simulink model "maglev"  (Simulink 9.1)
settings: Solver=ode45  StartTime=0.0  StopTime=9  MaxStep=T/10  RelTol=1e-3  EnableMultiTasking=on
StopFcn:
  | geragraficos
values from neighbouring files (symbols this model uses):
  dt = 0.001    [kalman_function.m]    (also in q6.m = 0.005)
  Gcd = 60*tf([1/alphae 1-1/alphae-exp(-tempo/(alphae*T))],[1 -exp(-tempo/(alphae*T))], tempo)    [q6.m]
  h_sig = 0.002/3    (= 0.000666666666667)    [q6.m]
  P0 = [0 0; 0 0]    [q6.m]
  x0 = [href;0]    [q6.m]
undefined symbols (not defined in the file or in its folder): sigbuilder_block
settings Model: Creator=cairo  LastModifiedBy=Avell
settings DataIOCC: LimitDataPoints=on  SignalLoggingSaveFormat=ModelDataLogs
settings OptimizationCC: ExpressionDepthLimit=2147483647  InitFltsAndDblsToZero=on
settings DebuggingCC: SaveWithParameterizedLinksMsg=none  SignalResolutionControl=TryResolveAllWithWarning  SolverPrmCheckMsg=warning  MultiTaskDSMMsg=warning  MultiTaskCondExecSysMsg=none  FcnCallInpInsideContextMsg=warning  StateNameClashWarn=warning
settings GRTTargetCC: TargetFcnLib=ansi_tfl_tmw.mat  GeneratePreprocessorConditionals=Disable all

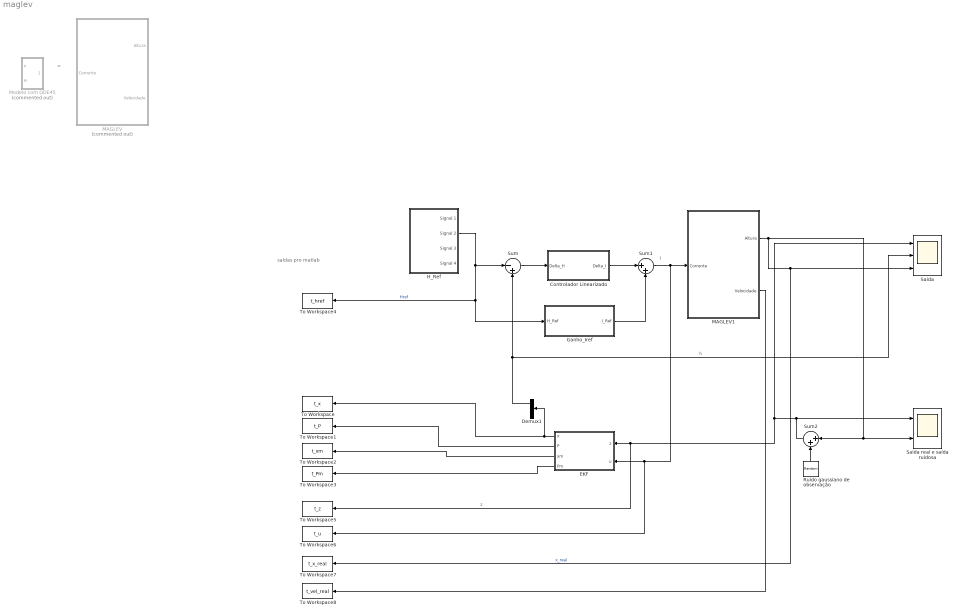
== system maglev ==
  note: saídas pro matlab
  note: =
  note: I
  Controlador Linearizado : Subsystem  mask(Controlador em avanço + termo integrador){}
  Demux1 : Demux  Outputs=2
  EKF : Subsystem
  Ganho_Iref : Subsystem  mask(Cálculo da corrente de referência (I_Ref) a partir da altura de referência (H_Ref)){Kb=0.12e-3, M=21.2e-3, g=9.8}
      mask prompts: Kb "Constante da bobina (Nm^2/A^2)"; M "Massa (kg)"; g "Gravidade (m/s^2)"
  H_Ref : Subsystem  Tag=STV Subsys  LoadFcn=sigbuilder_block('load');  StartFcn=sigbuilder_block('start');  StopFcn=sigbuilder_block('stop');  ClipboardFcn=sigbuilder_block('clipboard');  mask(Sigbuilder block){tuvar=[0:10]}
      mask help: Sigbuilder GUI
      mask init:
      | if ~strcmp(get_param(bdroot(gcbh),'SimulationStatus'),'stopped') tuvar = sigbuilder_block('maskInit'); end
      settings: CopyFcn=sigbuilder_block('copy');  DeleteFcn=sigbuilder_block('delete');  ModelCloseFcn=sigbuilder_block('modelClose');  PreSaveFcn=sigbuilder_block('preSave');  PauseFcn=sigbuilder_block('pause')  ContinueFcn=sigbuilder_block('continue')  NameChangeFcn=sigbuilder_block('namechange');  OpenFcn=sigbuilder_block('open',[0 0 1390.5 752.25 ]);  CloseFcn=sigbuilder_block('close');
      mask Display: plot(0, 0, 100, 100,[2, 2, 32, 32, 2], [68, 8, 8, 68, 68],[32, 2], [38, 38], [32, 19, 2],[53, 60, 44], [32, 17, 17, 2],[16, 16, 31, 31]);txt = getActiveGroup(gcbh);text(2, 100, txt,'verticalAlignment', 'top');
  MAGLEV : Subsystem  Commented=on  mask{Kb=0.12e-3, M=21.2e-3, g=9.8, x1_0=0.030, x2_0=0}
      mask prompts: Kb "Constante da bobina (Nm^2/A^2)"; M "Massa (kg)"; g "Gravidade (m/s^2)"; x1_0 "Altura inicial (m)"; x2_0 "Velocidade Inicial (m/s)"
      mask help: Modelo do Sistema de Levitação Magnética
      mask Display: image(imread('maglev_fig.jpg'),[0,0,350/2.5,525/2.5]);
  MAGLEV1 : Subsystem  mask{Kb=0.12e-3, M=21.2e-3, g=9.8, x1_0=0.030, x2_0=0}
      mask prompts: Kb "Constante da bobina (Nm^2/A^2)"; M "Massa (kg)"; g "Gravidade (m/s^2)"; x1_0 "Altura inicial (m)"; x2_0 "Velocidade Inicial (m/s)"
      mask help: Modelo do Sistema de Levitação Magnética
      mask Display: image(imread('maglev_fig.jpg'),[0,0,350/2.5,525/2.5]);
  Modelo com ODE45 : Subsystem  Commented=on
  Ruido gaussiano de observação : RandomNumber  Variance=h_sig^2  SampleTime=dt
  Saida : Scope  NumInputPorts=3
  Saida real e saída ruidosa : Scope  NumInputPorts=2
  Sum : Sum  Inputs=|-+
  Sum1 : Sum  Inputs=|++
  Sum2 : Sum  Inputs=|++
  To Workspace : ToWorkspace  VariableName=t_x  SaveFormat=Timeseries  SampleTime=-1
  To Workspace1 : ToWorkspace  VariableName=t_P  SaveFormat=Timeseries  SampleTime=-1
  To Workspace2 : ToWorkspace  VariableName=t_xm  SaveFormat=Timeseries  SampleTime=-1
  To Workspace3 : ToWorkspace  VariableName=t_Pm  SaveFormat=Timeseries  SampleTime=-1
  To Workspace4 : ToWorkspace  VariableName=t_href  SaveFormat=Timeseries  SampleTime=-1
  To Workspace5 : ToWorkspace  VariableName=t_z  SaveFormat=Timeseries  SampleTime=-1
  To Workspace6 : ToWorkspace  VariableName=t_u  SaveFormat=Timeseries  SampleTime=-1
  To Workspace7 : ToWorkspace  VariableName=t_x_real  SaveFormat=Timeseries  SampleTime=-1
  To Workspace8 : ToWorkspace  VariableName=t_vel_real  SaveFormat=Timeseries  SampleTime=-1
  wires:
  Ganho_Iref/1(I_Ref) -> Sum1/2
  Sum/1 -> Controlador Linearizado/1(Delta_H)
  Controlador Linearizado/1(Delta_I) -> Sum1/1
  H_Ref/2(Signal 2) -> Ganho_Iref/1(H_Ref), To Workspace4/1, Sum/1  "Href"
  Ruido gaussiano de observação/1 -> Sum2/2
  Sum2/1 -> To Workspace5/1, EKF/1(z), Saida/1, Saida real e saída ruidosa/1  "z"
  MAGLEV1/1(Altura) -> Saida real e saída ruidosa/2, Sum2/1, To Workspace7/1, Saida/3  "x_real"
  Sum1/1 -> To Workspace6/1, EKF/2(u), MAGLEV1/1(Corrente)
  EKF/1(x) -> To Workspace/1, Demux1/1
  Demux1/1 -> Saida/2, Sum/2  "h"
  EKF/2(P) -> To Workspace1/1
  EKF/3(xm) -> To Workspace2/1
  EKF/4(Pm) -> To Workspace3/1
  MAGLEV1/2(Velocidade) -> To Workspace8/1

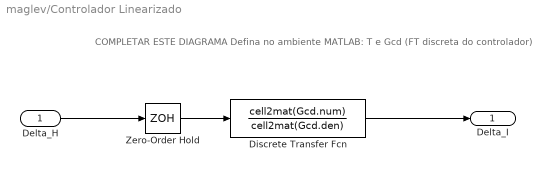
== system maglev/Controlador Linearizado ==
  note: COMPLETAR ESTE DIAGRAMA
      | Defina no ambiente MATLAB: T e Gcd (FT discreta do controlador)
  Delta_H : Inport
  Discrete Transfer Fcn : DiscreteTransferFcn  Numerator=cell2mat(Gcd.num)  Denominator=cell2mat(Gcd.den)
  Zero-Order Hold : ZeroOrderHold  SampleTime=dt
  Delta_I : Outport
  wires:
  Delta_H/1 -> Zero-Order Hold/1
  Discrete Transfer Fcn/1 -> Delta_I/1
  Zero-Order Hold/1 -> Discrete Transfer Fcn/1

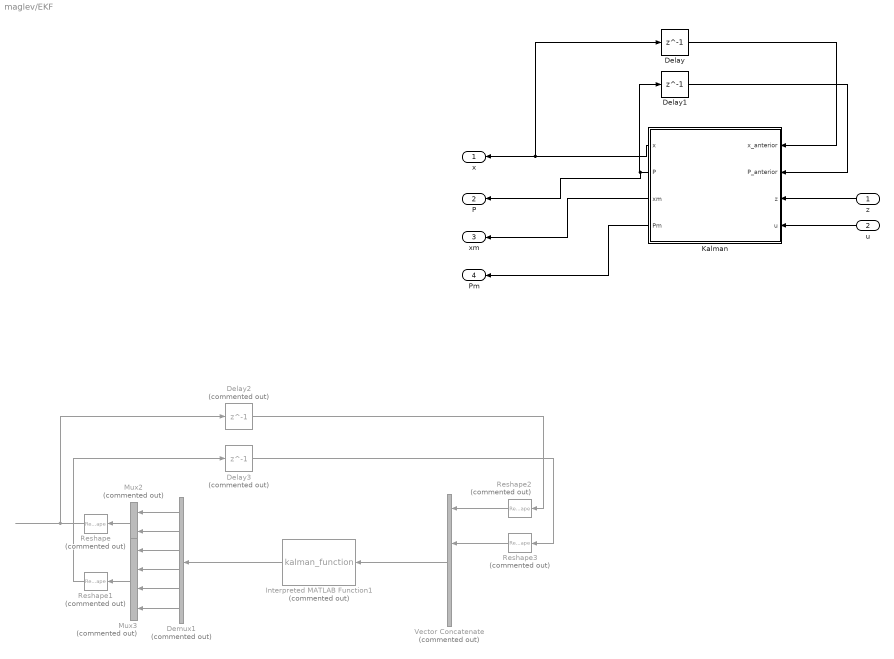
== system maglev/EKF ==
  z : Inport
  u : Inport  Port=2
  Delay : Delay  DelayLength=1  InitialCondition=x0
  Delay1 : Delay  DelayLength=1  InitialCondition=P0
  Delay2 : Delay  Commented=on  DelayLength=1  InitialCondition=x0
  Delay3 : Delay  Commented=on  DelayLength=1  InitialCondition=P0
  Demux1 : Demux  Commented=on  Outputs=6
  Interpreted MATLAB Function1 : MATLABFcn  Commented=on  MATLABFcn=kalman_function  OutputDimensions=6  Output1D=off
  Kalman : MATLAB Function  TreatAsAtomicUnit=on
  Mux2 : Mux  Commented=on  Inputs=2
  Mux3 : Mux  Commented=on
  Reshape : Reshape  Commented=on  OutputDimensionality=Customize  OutputDimensions=[2,1]
  Reshape1 : Reshape  Commented=on  OutputDimensionality=Customize  OutputDimensions=[2,2]
  Reshape2 : Reshape  Commented=on  OutputDimensions=[2,2]
  Reshape3 : Reshape  Commented=on  OutputDimensions=[2,2]
  Vector Concatenate : Concatenate  Commented=on  NumInputs=4
  x : Outport
  P : Outport  Port=2
  xm : Outport  Port=3
  Pm : Outport  Port=4
  wires:
  Kalman/1(x) -> x/1, Delay/1
  u/1 -> Kalman/4(u)
  Delay1/1 -> Kalman/2(P_anterior)
  Kalman/2(P) -> P/1, Delay1/1
  Delay/1 -> Kalman/1(x_anterior)
  z/1 -> Kalman/3(z)
  Interpreted MATLAB Function1/1 -> Demux1/1
  Demux1/1 -> Mux2/1
  Demux1/2 -> Mux2/2
  Mux2/1 -> Reshape/1
  Reshape/1 -> Delay2/1
  Demux1/3 -> Mux3/1
  Demux1/4 -> Mux3/2
  Demux1/5 -> Mux3/3
  Demux1/6 -> Mux3/4
  Mux3/1 -> Reshape1/1
  Reshape1/1 -> Delay3/1
  Delay2/1 -> Reshape2/1
  Reshape2/1 -> Vector Concatenate/1
  Reshape3/1 -> Vector Concatenate/2
  Delay3/1 -> Reshape3/1
  ? -> Vector Concatenate/3
  ? -> Vector Concatenate/4
  Vector Concatenate/1 -> Interpreted MATLAB Function1/1
  Kalman/3(xm) -> xm/1
  Kalman/4(Pm) -> Pm/1

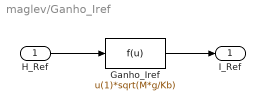
== system maglev/Ganho_Iref ==
  H_Ref : Inport
  Ganho_Iref : Fcn  Expr=u(1)*sqrt(M*g/Kb)
  I_Ref : Outport
  wires:
  Ganho_Iref/1 -> I_Ref/1
  H_Ref/1 -> Ganho_Iref/1

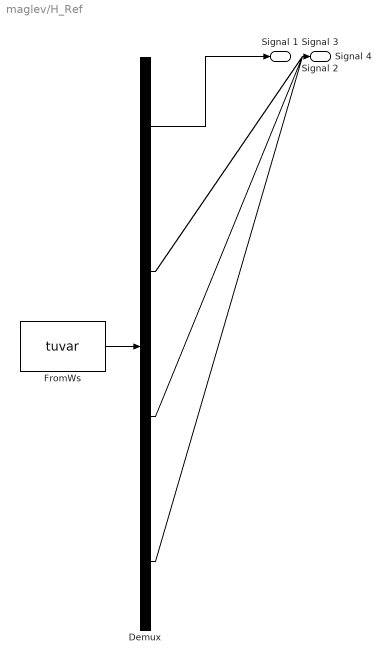
== system maglev/H_Ref ==
  Demux : Demux  Tag=STV Demux
  FromWs : FromWorkspace  Tag=STV FromWs  VariableName=tuvar  SampleTime=0  SigBuilderData=DataTag0  VnvData=DataTag1
      SigBuilderData=|
      | common.afterFinalStr = 'Extrapolate'
      | common.sampleTime = 0
      | dataSet.timeRange = [0 9]
      | dataSet.name = 'Group 1'
      | sbobj.Groups.Name = 'Group 1'
      | sbobj.Groups.Signals(1).Name = 'Signal 1'
      | sbobj.Groups.Signals(1).XData = [0 3 3 6 6 9]
      | sbobj.Groups.Signals(1).YData = [0.025 0.025 0.02 0.02 0.025 0.025]
      | sbobj.Groups.Signals(2).Name = 'Signal 2'
      | sbobj.Groups.Signals(2).XData = [0 0.222222222222 0.444444444444 0.666666666667 0.888888888889 1.11111111111 1.33333333333 1.55555555556 1.77777777778 2 2.22222222222 2.44444444444 2.66666666667 2.88888888889 3.11111111111 3.33333333333 3.55555555556 3.77777777778 4 4.22222222222 4.44444444444 4.66666666667 4.88888888889 5.11111111111 5.33333333333 5.55555555556 5.77777777778 6 6.22222222222 6.44444444444 6.66666666667 6.88888888889 7.11111111111 7.33333333333 7.55555555556 7.77777777778 8 8.22222222222 8.44444444444 8.66666666667 8.88888888889 9]
      | sbobj.Groups.Signals(2).YData = [0.0225 0.0257139380484 0.0274240387651 0.0268301270189 0.0242101007166 0.0207898992834 0.0181698729811 0.0175759612349 0.0192860619516 0.0225 0.0257139380484 0.0274240387651 0.0268301270189 0.0242101007166 0.0207898992834 0.0181698729811 0.0175759612349 0.0192860619516 0.0225 0.0257139380484 0.0274240387651 0.0268301270189 0.0242101007166 0.0207898992834 0.0181698729811 0.0175759612349 0.0192860619516 0.0225 0.0257139380484 0.0274240387651 0.0268301270189 0.0242101007166 0.0207898992834 0.0181698729811 0.0175759612349 0.0192860619516 0.0225 0.0257139380484 0.0274240387651 0.0268301270189 0.0242101007166 0.0225]
      | sbobj.Groups.Signals(3).Name = 'Signal 3'
      | sbobj.Groups.Signals(3).XData = [0 9]
      | sbobj.Groups.Signals(3).YData = [0.025 0.025]
      | sbobj.Groups.Signals(4).Name = 'Signal 4'
      | sbobj.Groups.Signals(4).XData = [0 2 2 4 4 6 6 8 8 9]
      | sbobj.Groups.Signals(4).YData = [0.02 0.03 0.02 0.03 0.02 0.03 0.02 0.03 0.02 0.025]
      | sbobj.Groups.TimeRange = [0 9]
  Signal 1 : Outport  Tag=STV Outport
  Signal 2 : Outport  Tag=STV Outport  Port=2
  Signal 3 : Outport  Tag=STV Outport  Port=3
  Signal 4 : Outport  Tag=STV Outport  Port=4
  wires:
  Demux/1 -> Signal 1/1
  FromWs/1 -> Demux/1
  Demux/2 -> Signal 2/1
  Demux/3 -> Signal 3/1
  Demux/4 -> Signal 4/1

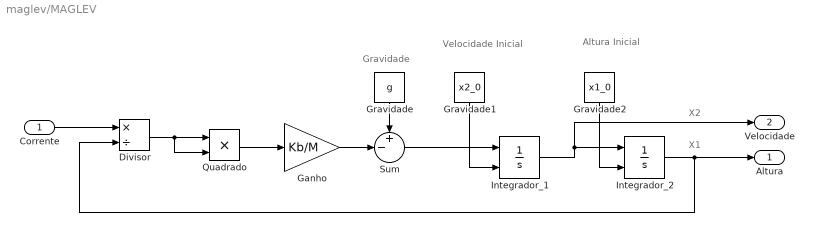
== system maglev/MAGLEV ==
  note: Gravidade
  note: X1
  note: X2
  note: Velocidade
      | Inicial
  note: Altura
      | Inicial
  Corrente : Inport
  Divisor : Product  Inputs=*/
  Ganho : Gain  Gain=Kb/M
  Gravidade : Constant  Value=g
  Gravidade1 : Constant  Value=x2_0
  Gravidade2 : Constant  Value=x1_0
  Integrador_1 : Integrator  InitialConditionSource=external  ZeroCross=off
  Integrador_2 : Integrator  InitialConditionSource=external  ZeroCross=off
  Quadrado : Product  Inputs=**
  Sum : Sum  Inputs=+-|
  Altura : Outport
  Velocidade : Outport  Port=2
  wires:
  Corrente/1 -> Divisor/1
  Divisor/1 -> Quadrado/1, Quadrado/2
  Quadrado/1 -> Ganho/1
  Ganho/1 -> Sum/2
  Gravidade/1 -> Sum/1
  Sum/1 -> Integrador_1/1
  Integrador_2/1 -> Divisor/2, Altura/1
  Gravidade1/1 -> Integrador_1/2
  Gravidade2/1 -> Integrador_2/2
  Integrador_1/1 -> Integrador_2/1, Velocidade/1

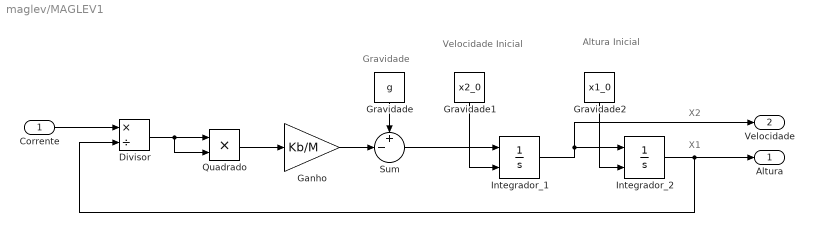
== system maglev/MAGLEV1 ==
  note: Gravidade
  note: X1
  note: X2
  note: Velocidade
      | Inicial
  note: Altura
      | Inicial
  Corrente : Inport
  Divisor : Product  Inputs=*/
  Ganho : Gain  Gain=Kb/M
  Gravidade : Constant  Value=g
  Gravidade1 : Constant  Value=x2_0
  Gravidade2 : Constant  Value=x1_0
  Integrador_1 : Integrator  InitialConditionSource=external  ZeroCross=off
  Integrador_2 : Integrator  InitialConditionSource=external  ZeroCross=off
  Quadrado : Product  Inputs=**
  Sum : Sum  Inputs=+-|
  Altura : Outport
  Velocidade : Outport  Port=2
  wires:
  Corrente/1 -> Divisor/1
  Divisor/1 -> Quadrado/1, Quadrado/2
  Quadrado/1 -> Ganho/1
  Ganho/1 -> Sum/2
  Gravidade/1 -> Sum/1
  Sum/1 -> Integrador_1/1
  Integrador_2/1 -> Divisor/2, Altura/1
  Gravidade1/1 -> Integrador_1/2
  Gravidade2/1 -> Integrador_2/2
  Integrador_1/1 -> Integrador_2/1, Velocidade/1

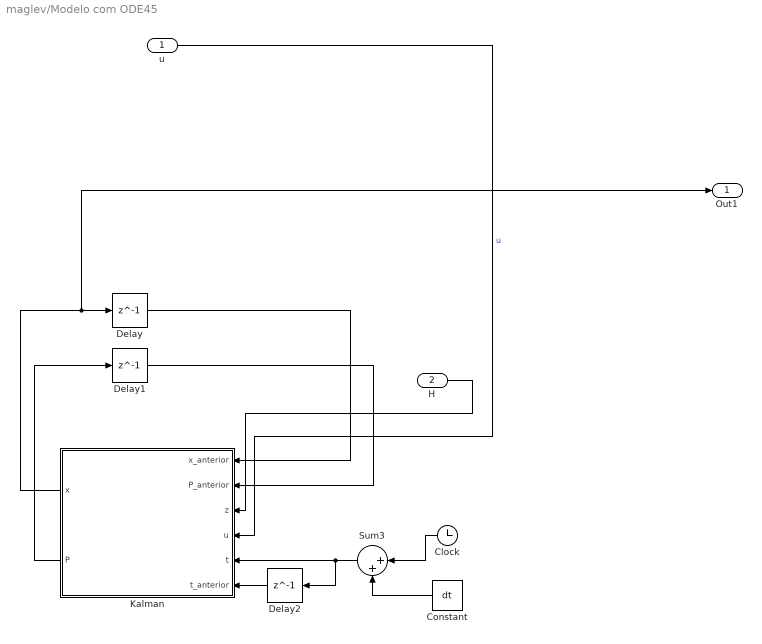
== system maglev/Modelo com ODE45 ==
  u : Inport
  H : Inport  Port=2
  Clock : Clock
  Constant : Constant  Value=dt  SampleTime=dt
  Delay : Delay  DelayLength=1  InitialCondition=x0
  Delay1 : Delay  DelayLength=1  InitialCondition=P0
  Delay2 : Delay  DelayLength=1  InitialCondition=0
  Kalman : MATLAB Function  TreatAsAtomicUnit=on
  Sum3 : Sum  Inputs=|++
  Out1 : Outport
  wires:
  Kalman/1(x) -> Out1/1, Delay/1
  Delay2/1 -> Kalman/6(t_anterior)
  Sum3/1 -> Delay2/1, Kalman/5(t)
  Constant/1 -> Sum3/2
  u/1 -> Kalman/4(u)  "u"
  Delay1/1 -> Kalman/2(P_anterior)
  Kalman/2(P) -> Delay1/1
  Delay/1 -> Kalman/1(x_anterior)
  H/1 -> Kalman/3(z)
  Clock/1 -> Sum3/1

== matlab function Modelo com ODE45/Kalman ==
  data: x_anterior input double; P_anterior input double; z input double; u input double; x output double; P output double; t input double; t_anterior input double
function [x, P]= fcn(x_anterior, P_anterior, z, u, t, t_anterior)
x = [0;0];
P = [0 0 ; 0 0];
dt = 0.001
%tspan = [t_anterior t];
tspan = [0 dt];
[T1,y] = ode45(@(t,x_anterior) nonlinear(t,x_anterior, u), tspan, x_anterior);
k1 = length(T1)
xm=(y(k1,1:2))'

x = xm
P = [0 0;0 0]

== matlab function EKF/Kalman ==
  data: x_anterior input double; P_anterior input double; z input double; u input double; x output double; P output double; xm output double; Pm output double
function [x, P,xm, Pm]= fcn(x_anterior, P_anterior, z, u)
%% Inicializa parâmetros
x = [0;0];
P = [0 0 ; 0 0];
g = 9.8;
kb = 0.12*10^(-3)
m = 21.2*10^(-3)
dt = 0.005;

% Define Q e R
Q = [(0.001/30)^2 0; 0 (0.001/30)^2]
R = (0.002/3)^2

%% Calcula A e H
% Calcula a matriz A linearizada em x_anterior e u
Ad = (eye(2)+dt*[0 1; 2*kb*u^2/(m*x_anterior(1)^3) 0]);

% Como nossa medida z é altura (mesma coisa de x(0)) H fica fácil
H = [1 0]

%% Propagação
xm = propaga_x()
Pm = Ad*P_anterior*(Ad') + Q

%% Atualização

K = Pm*(H')*inv(H*Pm*(H')+R)
xp = xm + K*(z-xm(1))
Pp = (eye(2) - K*H)*Pm



%% Propagação do novo x, com base em u e no valor antigo
   function x_menos = propaga_x
       % Resolver EDO
       [T1,y] = ode45(@(t,x_anterior) nonlinear(t,x_anterior, u), [0 dt], x_anterior); 
       % Pega o último valor
       x_menos=(y(length(T1),1:2))' 
   end

% %% Lineariza o sistema no ponto x_anterior e u. Retorna A discreto
%    function A_discreto = calcula_A_discreto
%        % Vamos linearizar em x_anterior e u:
%        Ac = [0 1; 2*kb*u^2/(m*x_anterior(1)^3) 0];
%        Bc = [0;-2*kb*u/(m*x_anterior(1)^2)];
%        Cc = [1 0];
%        Dc = 0;
%        % Discretizando o sistema fica:
%        discreteSys = ss(Ac,Bc,Cc,Dc,dt)
%        A_discreto = discreteSys.A
%    end

x = xp
P = Pp
end
